simulink model "SVPWMtrialsyedek"  (R2015b)
settings: Solver=VariableStepAuto  StartTime=0.0  StopTime=1  RelTol=1e-3
libraries: powerlib x1
(part 1 of 2)
settings Model: Creator=hakan  LastModifiedBy=hakan

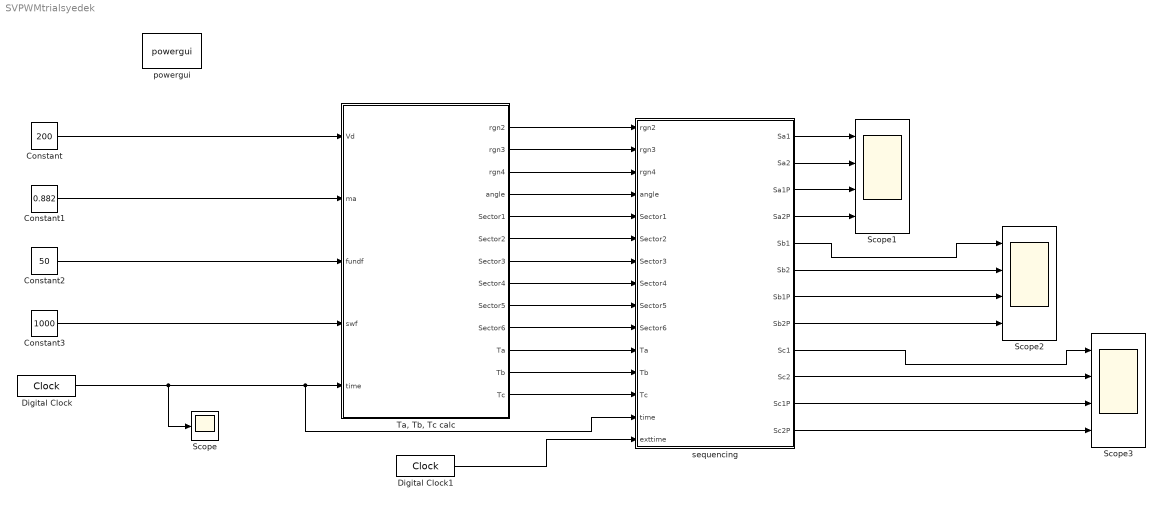
== system SVPWMtrialsyedek ==
  Constant : Constant  Value=200
  Constant1 : Constant  Value=0.882
  Constant2 : Constant  Value=50
  Constant3 : Constant  Value=1000
  Digital Clock : DigitalClock  SampleTime=0.001
  Digital Clock1 : DigitalClock  SampleTime=0.001
  Scope : Scope
  Scope1 : Scope  NumInputPorts=4
  Scope2 : Scope  NumInputPorts=4
  Scope3 : Scope  NumInputPorts=4
  "Ta, Tb, Tc calc" : MATLAB Function  TreatAsAtomicUnit=on
  powergui : powerlib/powergui  Priority=1  SimulationMode=Continuous  SolverType=Tustin/Backward Euler (TBE)  SampleTime=50e-6  frequency=60  SPID=off  DisableSnubberDevices=off  DisableRonSwitches=off  DisableVfSwitches=off  SwTol=0  DisplayEquations=off  Interpol=off  ExternalGateDelay=off  methode=off  Ts=10  FunctionMessages=off  echomessages=off  HookPort=off  EnableUseOfTLC=off  x0status=blocks  frequencyindice=60  Pbase=100e6  ErrMax=1e-4  Iterations=50  UnitsV=kV  UnitsW=MW  buscounter=0  RestoreLinks=warning  ResistiveCurrentMeasurement=off  Frange=[0:2:500]  Ylog=off  Xlog=on  ShowGrid=off  save=off  variable=ZData  structure=dutycycles  ZoomFFT=off  StartTime=0.0  cycles=1  DisplayStyle=1  fundamental=5000  FreqAxis=off  MaxFrequency=10000  frequencyindicesteady=1  RmsSteady=1  display=off
  sequencing : MATLAB Function  TreatAsAtomicUnit=on
  wires:
  Constant/1 -> "Ta, Tb, Tc calc"/1(Vd)
  Constant1/1 -> "Ta, Tb, Tc calc"/2(ma)
  Constant2/1 -> "Ta, Tb, Tc calc"/3(fundf)
  Constant3/1 -> "Ta, Tb, Tc calc"/4(swf)
  Digital Clock/1 -> sequencing/14(time), "Ta, Tb, Tc calc"/5(time), Scope/1
  "Ta, Tb, Tc calc"/1(rgn2) -> sequencing/1(rgn2)
  "Ta, Tb, Tc calc"/2(rgn3) -> sequencing/2(rgn3)
  "Ta, Tb, Tc calc"/3(rgn4) -> sequencing/3(rgn4)
  "Ta, Tb, Tc calc"/4(angle) -> sequencing/4(angle)
  "Ta, Tb, Tc calc"/5(Sector1) -> sequencing/5(Sector1)
  "Ta, Tb, Tc calc"/6(Sector2) -> sequencing/6(Sector2)
  "Ta, Tb, Tc calc"/7(Sector3) -> sequencing/7(Sector3)
  "Ta, Tb, Tc calc"/8(Sector4) -> sequencing/8(Sector4)
  "Ta, Tb, Tc calc"/10(Sector6) -> sequencing/10(Sector6)
  "Ta, Tb, Tc calc"/9(Sector5) -> sequencing/9(Sector5)
  "Ta, Tb, Tc calc"/11(Ta) -> sequencing/11(Ta)
  "Ta, Tb, Tc calc"/12(Tb) -> sequencing/12(Tb)
  "Ta, Tb, Tc calc"/13(Tc) -> sequencing/13(Tc)
  Digital Clock1/1 -> sequencing/15(exttime)
  sequencing/2(Sa2) -> Scope1/2
  sequencing/1(Sa1) -> Scope1/1
  sequencing/3(Sa1P) -> Scope1/3
  sequencing/4(Sa2P) -> Scope1/4
  sequencing/5(Sb1) -> Scope2/1
  sequencing/6(Sb2) -> Scope2/2
  sequencing/7(Sb1P) -> Scope2/3
  sequencing/8(Sb2P) -> Scope2/4
  sequencing/10(Sc2) -> Scope3/2
  sequencing/11(Sc1P) -> Scope3/3
  sequencing/12(Sc2P) -> Scope3/4
  sequencing/9(Sc1) -> Scope3/1

== matlab function SVPWMtrialsyedek/Ta, Tb, Tc calc ==
  data: rgn2 output; rgn3 output; rgn4 output; Vd input; ma input; fundf input; angle output; swf input; time input; Sector1 output; Sector2 output; Sector3 output; Sector4 output; Sector5 output; Sector6 output; Ta output; Tb output; Tc output
function [rgn2, rgn3, rgn4, angle, Sector1, Sector2, Sector3, Sector4, Sector5,Sector6, Ta, Tb, Tc] = fcn(Vd,ma,fundf, swf, time)
% this program works for magnitude of Vref is greater then Vd/3 meaning ma
% must be greater than 1/sqrt(3). for smaller ma's computation is a bit
% more tricky therefore it is omitted for simplicity for now. 
%#ok<*NASGU>
Vref = ma*Vd/sqrt(3); %magnitude of Vref
theta = 2*pi*fundf*time; %angle of Vref
angle = mod(theta, 2*pi);
Ts = 1/swf;
Ta = 0;
Tb = 0;
Tc = 0;
output = 0;
Sector1 = 0; Sector2 = 0; Sector3 = 0; Sector4= 0; Sector5 = 0; Sector6 = 0;
rgn2 = 0 ; rgn3 = 0; rgn4 = 0;
Sa1=0; Sa2=0; Sa1P=0; Sa2P=0; Sb1=0; Sb2=0; Sb1P=0; Sb2P=0; Sc1=0; Sc2=0; Sc1P=0; Sc2P=0;
%% Sector 1


if (mod(theta, 2*pi)<=pi/3)&&(mod(theta, 2*pi)>=0)  % sector 1

    n = 1;
    thetaprime = theta - (n-1)*pi/3;
    anglefrom3to2 = asin(1-1/(sqrt(3)*ma)); %leaving angle from region 3 to region 2
    anglefrom2to4 = pi/3 - anglefrom3to2; %leaving angle from region 2 to region 4
    if (mod(theta, 2*pi)<=anglefrom3to2) % then sector 1 region 3
        rgn3 = 1; rgn2= 0; rgn4=0;
        Ta = Ts*(2-2*ma*sin(pi/3+thetaprime));
        Tb = Ts*2*ma*sin(thetaprime);
        Tc = Ts*(2*ma*sin(pi/3-thetaprime)-1);        
    else if (mod(theta,2*pi)>=anglefrom3to2)&&(mod(theta,2*pi)<=anglefrom2to4) % then sector 1 region 2
            rgn3 = 0; rgn2= 1; rgn4=0;
            Ta = Ts*(1-2*ma*sin(thetaprime));
            Tb = Ts*(2*ma*sin(pi/3+thetaprime)-1);
            Tc = Ts*(1-2*ma*sin(pi/3-thetaprime));       
        else if (mod(theta,2*pi)>=anglefrom2to4) % then sector 1 region 4
               rgn3 = 0; rgn2= 0; rgn4=1;
               Ta = Ts*(2*ma*sin(thetaprime)-1);
               Tb = Ts*(2*ma*sin(pi/3-thetaprime));
               Tc = Ts*(2-2*ma*sin(pi/3+thetaprime));               
            end
        end
    end
    Sector1 = 1; Sector2 = 0; Sector3 = 0; Sector4= 0; Sector5 = 0; Sector6 = 0;
end
%% Sector 2


if (mod(theta, 2*pi)<=2*pi/3)&&(mod(theta, 2*pi)>=pi/3)  % sector 2
    
    n = 2;
    thetaprime = theta - (n-1)*pi/3;
    anglefrom3to2 = pi/3 + asin(1-1/(sqrt(3)*ma));
    anglefrom2to4 = pi/3 + pi/3 - anglefrom3to2;
    if (mod(theta, 2*pi)<=anglefrom3to2) % then sector 2 region 3
        rgn3 = 1; rgn2= 0; rgn4=0;
        Ta = Ts*(2-2*ma*sin(pi/3+thetaprime));
        Tb = Ts*2*ma*sin(thetaprime);
        Tc = Ts*(2*ma*sin(pi/3-thetaprime)-1); 
    else if (mod(theta,2*pi)>=anglefrom3to2)&&(mod(theta,2*pi)<=anglefrom2to4) % then sector 2 region 2
            rgn3 = 0; rgn2= 1; rgn4=0;
            Ta = Ts*(1-2*ma*sin(thetaprime));
            Tb = Ts*(2*ma*sin(pi/3+thetaprime)-1);
            Tc = Ts*(1-2*ma*sin(pi/3-thetaprime)); 
        else if (mod(theta,2*pi)>=anglefrom2to4) % then sector 2 region 4
               rgn3 = 0; rgn2= 0; rgn4=1;
               Ta = Ts*(2*ma*sin(thetaprime)-1);
               Tb = Ts*(2*ma*sin(pi/3-thetaprime));
               Tc = Ts*(2-2*ma*sin(pi/3+thetaprime)); 
            end
        end
    end
    Sector1 = 0; Sector2 = 1; Sector3 = 0; Sector4= 0; Sector5 = 0; Sector6 = 0;
end
%% Sector 3

if (mod(theta, 2*pi)<=pi)&&(mod(theta, 2*pi)>=2*pi/3)  % sector 3
    
    n = 3;
    thetaprime = theta - (n-1)*pi/3;
    anglefrom3to2 = 2*pi/3 + asin(1-1/(sqrt(3)*ma));
    anglefrom2to4 = 2*pi/3 + pi/3 - anglefrom3to2;
    if (mod(theta, 2*pi)<=anglefrom3to2) % then sector 3 region 3
        rgn3 = 1; rgn2= 0; rgn4=0;
        Ta = Ts*(2-2*ma*sin(pi/3+thetaprime));
        Tb = Ts*2*ma*sin(thetaprime);
        Tc = Ts*(2*ma*sin(pi/3-thetaprime)-1); 
    else if (mod(theta,2*pi)>=anglefrom3to2)&&(mod(theta,2*pi)<=anglefrom2to4) % then sector 3 region 2
            rgn3 = 0; rgn2= 1; rgn4=0;
            Ta = Ts*(1-2*ma*sin(thetaprime));
            Tb = Ts*(2*ma*sin(pi/3+thetaprime)-1);
            Tc = Ts*(1-2*ma*sin(pi/3-thetaprime)); 
        else if (mod(theta,2*pi)>=anglefrom2to4) % then sector 3 region 4
                rgn3 = 0; rgn2= 0; rgn4=1;
               Ta = Ts*(2*ma*sin(thetaprime)-1);
               Tb = Ts*(2*ma*sin(pi/3-thetaprime));
               Tc = Ts*(2-2*ma*sin(pi/3+thetaprime)); 
            end
        end
    end
    Sector1 = 0; Sector2 = 0; Sector3 = 1; Sector4= 0; Sector5 = 0; Sector6 = 0;
end

%% Sector 4


if (mod(theta, 2*pi)<=4*pi/3)&&(mod(theta, 2*pi)>=pi)  % sector 4
    

    n = 4;
    thetaprime = theta - (n-1)*pi/3;
    anglefrom3to2 = pi + asin(1-1/(sqrt(3)*ma));
    anglefrom2to4 = pi + pi/3 - anglefrom3to2;
    if (mod(theta, 2*pi)<=anglefrom3to2) % then sector 4 region 3
        rgn3 = 1; rgn2= 0; rgn4=0;
        Ta = Ts*(2-2*ma*sin(pi/3+thetaprime));
        Tb = Ts*2*ma*sin(thetaprime);
        Tc = Ts*(2*ma*sin(pi/3-thetaprime)-1); 
    else if (mod(theta,2*pi)>=anglefrom3to2)&&(mod(theta,2*pi)<=anglefrom2to4) % then sector 4 region 2
            rgn3 = 0; rgn2= 1; rgn4=0;
            Ta = Ts*(1-2*ma*sin(thetaprime));
            Tb = Ts*(2*ma*sin(pi/3+thetaprime)-1);
            Tc = Ts*(1-2*ma*sin(pi/3-thetaprime));
        else if (mod(theta,2*pi)>=anglefrom2to4) % then sector 4 region 4
                rgn3 = 0; rgn2= 0; rgn4=1;
               Ta = Ts*(2*ma*sin(thetaprime)-1);
               Tb = Ts*(2*ma*sin(pi/3-thetaprime));
               Tc = Ts*(2-2*ma*sin(pi/3+thetaprime)); 
            end
        end
    end
    Sector1 = 0; Sector2 = 0; Sector3 = 0; Sector4= 1; Sector5 = 0; Sector6 = 0;
end
%% Sector 5 

if (mod(theta, 2*pi)<=5*pi/3)&&(mod(theta, 2*pi)>=4*pi/3)  % sector 5
    
    n = 5;
    thetaprime = theta - (n-1)*pi/3;
    anglefrom3to2 = 4*pi/3 + asin(1-1/(sqrt(3)*ma));
    anglefrom2to4 = 4*pi/3 + pi/3 - anglefrom3to2;
    if (mod(theta, 2*pi)<=anglefrom3to2) % then sector 5 region 3
        rgn3 = 1; rgn2= 0; rgn4=0;
        Ta = Ts*(2-2*ma*sin(pi/3+thetaprime));
        Tb = Ts*2*ma*sin(thetaprime);
        Tc = Ts*(2*ma*sin(pi/3-thetaprime)-1); 
    else if (mod(theta,2*pi)>=anglefrom3to2)&&(mod(theta,2*pi)<=anglefrom2to4) % then sector 5 region 2
            rgn3 = 0; rgn2= 1; rgn4=0;
            Ta = Ts*(1-2*ma*sin(thetaprime));
            Tb = Ts*(2*ma*sin(pi/3+thetaprime)-1);
            Tc = Ts*(1-2*ma*sin(pi/3-thetaprime));
        else if (mod(theta,2*pi)>=anglefrom2to4) % then sector 5 region 4
               rgn3 = 0; rgn2= 0; rgn4=1;
               Ta = Ts*(2*ma*sin(thetaprime)-1);
               Tb = Ts*(2*ma*sin(pi/3-thetaprime));
               Tc = Ts*(2-2*ma*sin(pi/3+thetaprime)); 
            end
        end
    end
    Sector1 = 0; Sector2 = 0; Sector3 = 0; Sector4= 0; Sector5 = 1; Sector6 = 0;
end

%% Sector 6 

if (mod(theta, 2*pi)<=2*pi)&&(mod(theta, 2*pi)>=5*pi/3)  % sector 6
    
    n = 6;
    thetaprime = theta - (n-1)*pi/3;
    anglefrom3to2 = 5*pi/3 + asin(1-1/(sqrt(3)*ma));
    anglefrom2to4 = 5*pi/3 + pi/3 - anglefrom3to2;
    if (mod(theta, 2*pi)<=anglefrom3to2) % then sector 6 region 3
        rgn3 = 1; rgn2= 0; rgn4=0;
        Ta = Ts*(2-2*ma*sin(pi/3+thetaprime));
        Tb = Ts*2*ma*sin(thetaprime);
        Tc = Ts*(2*ma*sin(pi/3-thetaprime)-1); 
    else if (mod(theta,2*pi)>=anglefrom3to2)&&(mod(theta,2*pi)<=anglefrom2to4) % then sector 6 region 2
            rgn3 = 0; rgn2= 1; rgn4=0;
            Ta = Ts*(1-2*ma*sin(thetaprime));
            Tb = Ts*(2*ma*sin(pi/3+thetaprime)-1);
            Tc = Ts*(1-2*ma*sin(pi/3-thetaprime));
        else if (mod(theta,2*pi)>=anglefrom2to4) % then sector 6 region 4
               rgn3 = 0; rgn2= 0; rgn4=1;
               Ta = Ts*(2*ma*sin(thetaprime)-1);
               Tb = Ts*(2*ma*sin(pi/3-thetaprime));
               Tc = Ts*(2-2*ma*sin(pi/3+thetaprime)); 
            end
        end
    end
    Sector1 = 0; Sector2 = 0; Sector3 = 0; Sector4= 0; Sector5 = 0; Sector6 = 1;
end
%% Sequencing Part
% while(Sector1)
%     while(rgn3)
%         Sa1=0; Sa2=1; Sa1P=1; Sa2P=0;
%         Sb1=0; Sb2=0; Sb1P=1; Sb2P=1; 
%         Sc1=0; Sc2=0; Sc1P=1; Sc2P=1;
%         pause(Tc/4);
%         Sa1=1; Sa2=1; Sa1P=0; Sa2P=0;
%         Sb1=0; Sb2=0; Sb1P=1; Sb2P=1; 
%         Sc1=0; Sc2=0; Sc1P=1; Sc2P=1;
%         pause(Tb/2);
%         Sa1=1; Sa2=1; Sa1P=0; Sa2P=0;
%         Sb1=0; Sb2=1; Sb1P=1; Sb2P=0; 
%         Sc1=0; Sc2=0; Sc1P=1; Sc2P=1;
%         pause(Ta/2);
%         Sa1=1; Sa2=1; Sa1P=0; Sa2P=0;
%         Sb1=0; Sb2=1; Sb1P=1; Sb2P=0; 
%         Sc1=0; Sc2=1; Sc1P=1; Sc2P=0;
%         pause(Tc/2);
%         Sa1=1; Sa2=1; Sa1P=0; Sa2P=0;
%         Sb1=0; Sb2=1; Sb1P=1; Sb2P=0; 
%         Sc1=0; Sc2=0; Sc1P=1; Sc2P=1;
%         pause(Ta/2);
%         Sa1=1; Sa2=1; Sa1P=0; Sa2P=0;
%         Sb1=0; Sb2=0; Sb1P=1; Sb2P=1; 
%         Sc1=0; Sc2=0; Sc1P=1; Sc2P=1;
%         pause(Tb/2);
%         Sa1=0; Sa2=1; Sa1P=1; Sa2P=0;
%         Sb1=0; Sb2=0; Sb1P=1; Sb2P=1; 
%         Sc1=0; Sc2=0; Sc1P=1; Sc2P=1;
%         pause(Tc/4);        
%     end
%     while(rgn2)
%         if angle<= pi/6 % then 2a
%             Sa1=0; Sa2=1; Sa1P=1; Sa2P=0;
%             Sb1=0; Sb2=0; Sb1P=1; Sb2P=1; 
%             Sc1=0; Sc2=0; Sc1P=1; Sc2P=1;
%             pause(Tc/4);
%             Sa1=0; Sa2=1; Sa1P=1; Sa2P=0;
%             Sb1=0; Sb2=1; Sb1P=1; Sb2P=0; 
%             Sc1=0; Sc2=0; Sc1P=1; Sc2P=1;
%             pause(Tb/2);
%             Sa1=1; Sa2=1; Sa1P=0; Sa2P=0;
%             Sb1=0; Sb2=1; Sb1P=1; Sb2P=0; 
%             Sc1=0; Sc2=0; Sc1P=1; Sc2P=1;       
%             pause(Ta/2);
%             Sa1=1; Sa2=1; Sa1P=0; Sa2P=0;
%             Sb1=0; Sb2=1; Sb1P=1; Sb2P=0; 
%             Sc1=0; Sc2=1; Sc1P=1; Sc2P=0;
%             pause(Tc/2);
%             Sa1=1; Sa2=1; Sa1P=0; Sa2P=0;
%             Sb1=0; Sb2=1; Sb1P=1; Sb2P=0; 
%             Sc1=0; Sc2=0; Sc1P=1; Sc2P=1;
%             pause(Ta/2);
%             Sa1=0; Sa2=1; Sa1P=1; Sa2P=0;
%             Sb1=0; Sb2=1; Sb1P=1; Sb2P=0; 
%             Sc1=0; Sc2=0; Sc1P=1; Sc2P=1;
%             pause(Tb/2);
%             Sa1=0; Sa2=1; Sa1P=1; Sa2P=0;
%             Sb1=0; Sb2=0; Sb1P=1; Sb2P=1; 
%             Sc1=0; Sc2=0; Sc1P=1; Sc2P=1;
%             pause(Tc/4);        
%         end
%         if angle>= pi/6 % then 2b
%             Sa1=0; Sa2=1; Sa1P=1; Sa2P=0;
%             Sb1=0; Sb2=1; Sb1P=1; Sb2P=0; 
%             Sc1=0; Sc2=0; Sc1P=1; Sc2P=1;
%             pause(Tc/4);
%             Sa1=1; Sa2=1; Sa1P=0; Sa2P=0;
%             Sb1=0; Sb2=1; Sb1P=1; Sb2P=0; 
%             Sc1=0; Sc2=0; Sc1P=1; Sc2P=1;
%             pause(Tb/2);
%             Sa1=1; Sa2=1; Sa1P=0; Sa2P=0;
%             Sb1=0; Sb2=1; Sb1P=1; Sb2P=0; 
%             Sc1=0; Sc2=1; Sc1P=1; Sc2P=0;
%             pause(Ta/2);
%             Sa1=1; Sa2=1; Sa1P=0; Sa2P=0;
%             Sb1=1; Sb2=1; Sb1P=0; Sb2P=0; 
%             Sc1=0; Sc2=1; Sc1P=1; Sc2P=0;
%             pause(Tc/2);
%             Sa1=1; Sa2=1; Sa1P=0; Sa2P=0;
%             Sb1=0; Sb2=1; Sb1P=1; Sb2P=0; 
%             Sc1=0; Sc2=1; Sc1P=1; Sc2P=0;
%             pause(Ta/2);
%             Sa1=1; Sa2=1; Sa1P=0; Sa2P=0;
%             Sb1=0; Sb2=1; Sb1P=1; Sb2P=0; 
%             Sc1=0; Sc2=0; Sc1P=1; Sc2P=1;
%             pause(Tb/2);
%             Sa1=0; Sa2=1; Sa1P=1; Sa2P=0;
%             Sb1=0; Sb2=1; Sb1P=1; Sb2P=0; 
%             Sc1=0; Sc2=0; Sc1P=1; Sc2P=1;
%             pause(Tc/4);
%         end
%     end
%     while(rgn4)
%         Sa1=0; Sa2=1; Sa1P=1; Sa2P=0;
%         Sb1=0; Sb2=1; Sb1P=1; Sb2P=0;
%         Sc1=0; Sc2=0; Sc1P=1; Sc2P=1;
%         pause(Tc/4);
%         Sa1=1; Sa2=1; Sa1P=0; Sa2P=0;
%         Sb1=0; Sb2=1; Sb1P=1; Sb2P=0;
%         Sc1=0; Sc2=0; Sc1P=1; Sc2P=1;        
%         pause(Tb/2);        
%         Sa1=1; Sa2=1; Sa1P=0; Sa2P=0;
%         Sb1=1; Sb2=1; Sb1P=0; Sb2P=0;
%         Sc1=0; Sc2=0; Sc1P=1; Sc2P=1;
%         pause(Ta/2);
%         Sa1=1; Sa2=1; Sa1P=0; Sa2P=0;
%         Sb1=1; Sb2=1; Sb1P=0; Sb2P=0;
%         Sc1=0; Sc2=1; Sc1P=1; Sc2P=0;
%         pause(Tc/2);
%         Sa1=1; Sa2=1; Sa1P=0; Sa2P=0;
%         Sb1=1; Sb2=1; Sb1P=0; Sb2P=0;
%         Sc1=0; Sc2=0; Sc1P=1; Sc2P=1;
%         pause(Ta/2);        
%         Sa1=1; Sa2=1; Sa1P=0; Sa2P=0;
%         Sb1=0; Sb2=1; Sb1P=1; Sb2P=0;
%         Sc1=0; Sc2=0; Sc1P=1; Sc2P=1;        
%         pause(Tb/2);
%         Sa1=0; Sa2=1; Sa1P=1; Sa2P=0;
%         Sb1=0; Sb2=1; Sb1P=1; Sb2P=0;
%         Sc1=0; Sc2=0; Sc1P=1; Sc2P=1;
%         pause(Tc/4);
%     end
% end
% while(Sector2)
%     while(rgn3)        
%         Sa1=0; Sa2=1; Sa1P=1; Sa2P=0;
%         Sb1=0; Sb2=1; Sb1P=1; Sb2P=0;
%         Sc1=0; Sc2=0; Sc1P=1; Sc2P=1;
%         pause(Tc/4);
%         Sa1=0; Sa2=1; Sa1P=1; Sa2P=0;
%         Sb1=1; Sb2=1; Sb1P=0; Sb2P=0;
%         Sc1=0; Sc2=0; Sc1P=1; Sc2P=1;
%         pause(Tb/2);
%         Sa1=1; Sa2=1; Sa1P=0; Sa2P=0;
%         Sb1=1; Sb2=1; Sb1P=0; Sb2P=0;
%         Sc1=0; Sc2=0; Sc1P=1; Sc2P=1;
%         pause(Ta/2);
%         Sa1=1; Sa2=1; Sa1P=0; Sa2P=0;
%         Sb1=1; Sb2=1; Sb1P=0; Sb2P=0;
%         Sc1=0; Sc2=1; Sc1P=1; Sc2P=0;       
%         pause(Tc/2);
%         Sa1=1; Sa2=1; Sa1P=0; Sa2P=0;
%         Sb1=1; Sb2=1; Sb1P=0; Sb2P=0;
%         Sc1=0; Sc2=0; Sc1P=1; Sc2P=1;
%         pause(Ta/2);
%         Sa1=0; Sa2=1; Sa1P=1; Sa2P=0;
%         Sb1=1; Sb2=1; Sb1P=0; Sb2P=0;
%         Sc1=0; Sc2=0; Sc1P=1; Sc2P=1;
%         pause(Tb/2);
%         Sa1=0; Sa2=1; Sa1P=1; Sa2P=0;
%         Sb1=0; Sb2=1; Sb1P=1; Sb2P=0;
%         Sc1=0; Sc2=0; Sc1P=1; Sc2P=1;
%         pause(Tc/4);       
%     end
%     while(rgn2)
%         if angle<=pi/2 %then 2a
%             Sa1=0; Sa2=1; Sa1P=1; Sa2P=0;
%             Sb1=0; Sb2=1; Sb1P=1; Sb2P=0;
%             Sc1=0; Sc2=0; Sc1P=1; Sc2P=1;
%             pause(Tc/4);
%             Sa1=0; Sa2=1; Sa1P=1; Sa2P=0;
%             Sb1=1; Sb2=1; Sb1P=0; Sb2P=0;
%             Sc1=0; Sc2=0; Sc1P=1; Sc2P=1;
%             pause(Tb/2);
%             Sa1=0; Sa2=1; Sa1P=1; Sa2P=0;
%             Sb1=1; Sb2=1; Sb1P=0; Sb2P=0;
%             Sc1=0; Sc2=1; Sc1P=1; Sc2P=0;
%             pause(Ta/2);
%             Sa1=1; Sa2=1; Sa1P=0; Sa2P=0;
%             Sb1=1; Sb2=1; Sb1P=0; Sb2P=0;
%             Sc1=0; Sc2=1; Sc1P=1; Sc2P=0;            
%             pause(Tc/2);
%             Sa1=0; Sa2=1; Sa1P=1; Sa2P=0;
%             Sb1=1; Sb2=1; Sb1P=0; Sb2P=0;
%             Sc1=0; Sc2=1; Sc1P=1; Sc2P=0;
%             pause(Ta/2);
%             Sa1=0; Sa2=1; Sa1P=1; Sa2P=0;
%             Sb1=1; Sb2=1; Sb1P=0; Sb2P=0;
%             Sc1=0; Sc2=0; Sc1P=1; Sc2P=1;
%             pause(Tb/2);
%             Sa1=0; Sa2=1; Sa1P=1; Sa2P=0;
%             Sb1=0; Sb2=1; Sb1P=1; Sb2P=0;
%             Sc1=0; Sc2=0; Sc1P=1; Sc2P=1;
%             pause(Tc/4);
%         end
%         if angle>=pi/2 %then 2b
%             Sa1=0; Sa2=0; Sa1P=1; Sa2P=1;
%             Sb1=0; Sb2=1; Sb1P=1; Sb2P=0;
%             Sc1=0; Sc2=0; Sc1P=1; Sc2P=1;
%             pause(Tc/4);
%             Sa1=0; Sa2=1; Sa1P=1; Sa2P=0;
%             Sb1=0; Sb2=1; Sb1P=1; Sb2P=0;
%             Sc1=0; Sc2=0; Sc1P=1; Sc2P=1;
%             pause(Tb/2);
%             Sa1=0; Sa2=1; Sa1P=1; Sa2P=0;
%             Sb1=1; Sb2=1; Sb1P=0; Sb2P=0;
%             Sc1=0; Sc2=0; Sc1P=1; Sc2P=1;
%             pause(Ta/2);
%             Sa1=0; Sa2=1; Sa1P=1; Sa2P=0;
%             Sb1=1; Sb2=1; Sb1P=0; Sb2P=0;
%             Sc1=0; Sc2=1; Sc1P=1; Sc2P=0;
%             pause(Tc/2);
%             Sa1=0; Sa2=1; Sa1P=1; Sa2P=0;
%             Sb1=1; Sb2=1; Sb1P=0; Sb2P=0;
%             Sc1=0; Sc2=0; Sc1P=1; Sc2P=1;
%             pause(Ta/2);
%             Sa1=0; Sa2=1; Sa1P=1; Sa2P=0;
%             Sb1=0; Sb2=1; Sb1P=1; Sb2P=0;
%             Sc1=0; Sc2=0; Sc1P=1; Sc2P=1;
%             pause(Tb/2);
%             Sa1=0; Sa2=0; Sa1P=1; Sa2P=1;
%             Sb1=0; Sb2=1; Sb1P=1; Sb2P=0;
%             Sc1=0; Sc2=0; Sc1P=1; Sc2P=1;
%             pause(Tc/4);           
%         end
%     end
%     while(rgn4)
%         Sa1=0; Sa2=0; Sa1P=1; Sa2P=1;
%         Sb1=0; Sb2=1; Sb1P=1; Sb2P=0;
%         Sc1=0; Sc2=0; Sc1P=1; Sc2P=1;
%         pause(Tc/4);
%         Sa1=0; Sa2=0; Sa1P=1; Sa2P=1;
%         Sb1=1; Sb2=1; Sb1P=0; Sb2P=0;
%         Sc1=0; Sc2=0; Sc1P=1; Sc2P=1;
%         pause(Tb/2);
%         Sa1=0; Sa2=1; Sa1P=1; Sa2P=0;
%         Sb1=1; Sb2=1; Sb1P=0; Sb2P=0;
%         Sc1=0; Sc2=0; Sc1P=1; Sc2P=1;
%         pause(Ta/2);
%         Sa1=0; Sa2=1; Sa1P=1; Sa2P=0;
%         Sb1=1; Sb2=1; Sb1P=0; Sb2P=0;
%         Sc1=0; Sc2=1; Sc1P=1; Sc2P=0;
%         pause(Tc/2); 
%         Sa1=0; Sa2=1; Sa1P=1; Sa2P=0;
%         Sb1=1; Sb2=1; Sb1P=0; Sb2P=0;
%         Sc1=0; Sc2=0; Sc1P=1; Sc2P=1;
%         pause(Ta/2);
%         Sa1=0; Sa2=0; Sa1P=1; Sa2P=1;
%         Sb1=1; Sb2=1; Sb1P=0; Sb2P=0;
%         Sc1=0; Sc2=0; Sc1P=1; Sc2P=1;
%         pause(Tb/2);
%         Sa1=0; Sa2=0; Sa1P=1; Sa2P=1;
%         Sb1=0; Sb2=1; Sb1P=1; Sb2P=0;
%         Sc1=0; Sc2=0; Sc1P=1; Sc2P=1;
%         pause(Tc/4);
%         
%     end
% 
% end
% while(Sector3)
%     while(rgn3)
%         Sa1=0; Sa2=0; Sa1P=1; Sa2P=1;
%         Sb1=0; Sb2=1; Sb1P=1; Sb2P=0;
%         Sc1=0; Sc2=0; Sc1P=1; Sc2P=1;
%         pause(Tc/4);
%         Sa1=0; Sa2=0; Sa1P=1; Sa2P=1;
%         Sb1=1; Sb2=1; Sb1P=0; Sb2P=0;
%         Sc1=0; Sc2=0; Sc1P=1; Sc2P=1;
%         pause(Tb/2);
%         Sa1=0; Sa2=0; Sa1P=1; Sa2P=1;
%         Sb1=1; Sb2=1; Sb1P=0; Sb2P=0;
%         Sc1=0; Sc2=1; Sc1P=1; Sc2P=0;
%         pause(Ta/2);
%         Sa1=0; Sa2=1; Sa1P=1; Sa2P=0;
%         Sb1=1; Sb2=1; Sb1P=0; Sb2P=0;
%         Sc1=0; Sc2=1; Sc1P=1; Sc2P=0;
%         pause(Tc/2);
%         Sa1=0; Sa2=0; Sa1P=1; Sa2P=1;
%         Sb1=1; Sb2=1; Sb1P=0; Sb2P=0;
%         Sc1=0; Sc2=1; Sc1P=1; Sc2P=0;
%         pause(Ta/2);
%         Sa1=0; Sa2=0; Sa1P=1; Sa2P=1;
%         Sb1=1; Sb2=1; Sb1P=0; Sb2P=0;
%         Sc1=0; Sc2=0; Sc1P=1; Sc2P=1;
%         pause(Tb/2);
%         Sa1=0; Sa2=0; Sa1P=1; Sa2P=1;
%         Sb1=0; Sb2=1; Sb1P=1; Sb2P=0;
%         Sc1=0; Sc2=0; Sc1P=1; Sc2P=1;
%         pause(Tc/4);        
%     end
%     while(rgn2)
%         if angle<=5*pi/6 %then 2a
%             Sa1=0; Sa2=0; Sa1P=1; Sa2P=1;
%             Sb1=0; Sb2=1; Sb1P=1; Sb2P=0;
%             Sc1=0; Sc2=0; Sc1P=1; Sc2P=1;
%             pause(Tc/4);
%             Sa1=0; Sa2=0; Sa1P=1; Sa2P=1;
%             Sb1=0; Sb2=1; Sb1P=1; Sb2P=0;
%             Sc1=0; Sc2=1; Sc1P=1; Sc2P=0;
%             pause(Tb/2);
%             Sa1=0; Sa2=0; Sa1P=1; Sa2P=1;
%             Sb1=1; Sb2=1; Sb1P=0; Sb2P=0;
%             Sc1=0; Sc2=1; Sc1P=1; Sc2P=0;
%             pause(Ta/2);
%             Sa1=0; Sa2=0; Sa1P=1; Sa2P=1;
%             Sb1=1; Sb2=1; Sb1P=0; Sb2P=0;
%             Sc1=0; Sc2=0; Sc1P=1; Sc2P=1;
%             pause(Tc/2);
%             Sa1=0; Sa2=0; Sa1P=1; Sa2P=1;
%             Sb1=1; Sb2=1; Sb1P=0; Sb2P=0;
%             Sc1=0; Sc2=1; Sc1P=1; Sc2P=0;
%             pause(Ta/2);
%             Sa1=0; Sa2=0; Sa1P=1; Sa2P=1;
%             Sb1=0; Sb2=1; Sb1P=1; Sb2P=0;
%             Sc1=0; Sc2=1; Sc1P=1; Sc2P=0;
%             pause(Tb/2);
%             Sa1=0; Sa2=0; Sa1P=1; Sa2P=1;
%             Sb1=0; Sb2=1; Sb1P=1; Sb2P=0;
%             Sc1=0; Sc2=0; Sc1P=1; Sc2P=1;
%             pause(Tc/4);           
%         end
%         if angle>=5*pi/6 %then 2b
%             Sa1=0; Sa2=0; Sa1P=1; Sa2P=1;
%             Sb1=0; Sb2=1; Sb1P=1; Sb2P=0;
%             Sc1=0; Sc2=1; Sc1P=1; Sc2P=0;
%             pause(Tc/4);
%             Sa1=0; Sa2=0; Sa1P=1; Sa2P=1;
%             Sb1=1; Sb2=1; Sb1P=0; Sb2P=0;
%             Sc1=0; Sc2=1; Sc1P=1; Sc2P=0;
%             pause(Tb/2);
%             Sa1=0; Sa2=1; Sa1P=1; Sa2P=0;
%             Sb1=1; Sb2=1; Sb1P=0; Sb2P=0;
%             Sc1=0; Sc2=1; Sc1P=1; Sc2P=0;
%             pause(Ta/2);
%             Sa1=0; Sa2=1; Sa1P=1; Sa2P=0;
%             Sb1=1; Sb2=1; Sb1P=0; Sb2P=0;
%             Sc1=1; Sc2=1; Sc1P=0; Sc2P=0;
%             pause(Tc/2);
%             Sa1=0; Sa2=1; Sa1P=1; Sa2P=0;
%             Sb1=1; Sb2=1; Sb1P=0; Sb2P=0;
%             Sc1=0; Sc2=1; Sc1P=1; Sc2P=0;
%             pause(Ta/2);
%             Sa1=0; Sa2=0; Sa1P=1; Sa2P=1;
%             Sb1=1; Sb2=1; Sb1P=0; Sb2P=0;
%             Sc1=0; Sc2=1; Sc1P=1; Sc2P=0;
%             pause(Tb/2);
%             Sa1=0; Sa2=0; Sa1P=1; Sa2P=1;
%             Sb1=0; Sb2=1; Sb1P=1; Sb2P=0;
%             Sc1=0; Sc2=1; Sc1P=1; Sc2P=0;
%             pause(Tc/4);            
%         end
%     end
%     while(rgn4)
%         Sa1=0; Sa2=0; Sa1P=1; Sa2P=1;
%         Sb1=0; Sb2=1; Sb1P=1; Sb2P=0;
%         Sc1=0; Sc2=1; Sc1P=1; Sc2P=0;
%         pause(Tc/4);
%         Sa1=0; Sa2=0; Sa1P=1; Sa2P=1;
%         Sb1=1; Sb2=1; Sb1P=0; Sb2P=0;
%         Sc1=0; Sc2=1; Sc1P=1; Sc2P=0;
%         pause(Tb/2);
%         Sa1=0; Sa2=0; Sa1P=1; Sa2P=1;
%         Sb1=1; Sb2=1; Sb1P=0; Sb2P=0;
%         Sc1=1; Sc2=1; Sc1P=0; Sc2P=0;
%         pause(Ta/2);
%         Sa1=0; Sa2=1; Sa1P=1; Sa2P=0;
%         Sb1=1; Sb2=1; Sb1P=0; Sb2P=0;
%         Sc1=1; Sc2=1; Sc1P=0; Sc2P=0;
%         pause(Tc/2);
%         Sa1=0; Sa2=0; Sa1P=1; Sa2P=1;
%         Sb1=1; Sb2=1; Sb1P=0; Sb2P=0;
%         Sc1=1; Sc2=1; Sc1P=0; Sc2P=0;
%         pause(Ta/2);
%         Sa1=0; Sa2=0; Sa1P=1; Sa2P=1;
%         Sb1=1; Sb2=1; Sb1P=0; Sb2P=0;
%         Sc1=0; Sc2=1; Sc1P=1; Sc2P=0;
%         pause(Tb/2);
%         Sa1=0; Sa2=0; Sa1P=1; Sa2P=1;
%         Sb1=0; Sb2=1; Sb1P=1; Sb2P=0;
%         Sc1=0; Sc2=1; Sc1P=1; Sc2P=0;
%         pause(Tc/4);
%     end
% end
% while(Sector4)
%     while(rgn3)        
%         Sa1=0; Sa2=1; Sa1P=1; Sa2P=0;
%         Sb1=1; Sb2=1; Sb1P=0; Sb2P=0;
%         Sc1=1; Sc2=1; Sc1P=0; Sc2P=0;
%         pause(Tc/4);
%         Sa1=0; Sa2=0; Sa1P=1; Sa2P=1;
%         Sb1=1; Sb2=1; Sb1P=0; Sb2P=0;
%         Sc1=1; Sc2=1; Sc1P=0; Sc2P=0;
%         pause(Tb/2);
%         Sa1=0; Sa2=0; Sa1P=1; Sa2P=1;
%         Sb1=0; Sb2=1; Sb1P=1; Sb2P=0;
%         Sc1=1; Sc2=1; Sc1P=0; Sc2P=0;
%         pause(Ta/2);
%         Sa1=0; Sa2=0; Sa1P=1; Sa2P=1;
%         Sb1=0; Sb2=1; Sb1P=1; Sb2P=0;
%         Sc1=0; Sc2=1; Sc1P=1; Sc2P=0;
%         pause(Tc/2);
%         Sa1=0; Sa2=0; Sa1P=1; Sa2P=1;
%         Sb1=0; Sb2=1; Sb1P=1; Sb2P=0;
%         Sc1=1; Sc2=1; Sc1P=0; Sc2P=0;
%         pause(Ta/2);
%         Sa1=0; Sa2=0; Sa1P=1; Sa2P=1;
%         Sb1=1; Sb2=1; Sb1P=0; Sb2P=0;
%         Sc1=1; Sc2=1; Sc1P=0; Sc2P=0;
%         pause(Tb/2);
%         Sa1=0; Sa2=1; Sa1P=1; Sa2P=0;
%         Sb1=1; Sb2=1; Sb1P=0; Sb2P=0;
%         Sc1=1; Sc2=1; Sc1P=0; Sc2P=0;
%         pause(Tc/4);
%     end
%     while(rgn2)
%         if angle<=7*pi/6 %then 2a
%             Sa1=0; Sa2=1; Sa1P=1; Sa2P=0;
%             Sb1=1; Sb2=1; Sb1P=0; Sb2P=0;
%             Sc1=1; Sc2=1; Sc1P=0; Sc2P=0;
%             pause(Tc/4);
%             Sa1=0; Sa2=1; Sa1P=1; Sa2P=0;
%             Sb1=0; Sb2=1; Sb1P=1; Sb2P=0;
%             Sc1=1; Sc2=1; Sc1P=0; Sc2P=0;
%             pause(Tb/2);
%             Sa1=0; Sa2=0; Sa1P=1; Sa2P=1;
%             Sb1=0; Sb2=1; Sb1P=1; Sb2P=0;
%             Sc1=1; Sc2=1; Sc1P=0; Sc2P=0;
%             pause(Ta/2);
%             Sa1=0; Sa2=0; Sa1P=1; Sa2P=1;
%             Sb1=0; Sb2=1; Sb1P=1; Sb2P=0;
%             Sc1=0; Sc2=1; Sc1P=1; Sc2P=0;
%             pause(Tc/2);
%             Sa1=0; Sa2=0; Sa1P=1; Sa2P=1;
%             Sb1=0; Sb2=1; Sb1P=1; Sb2P=0;
%             Sc1=1; Sc2=1; Sc1P=0; Sc2P=0;
%             pause(Ta/2);
%             Sa1=0; Sa2=1; Sa1P=1; Sa2P=0;
%             Sb1=0; Sb2=1; Sb1P=1; Sb2P=0;
%             Sc1=1; Sc2=1; Sc1P=0; Sc2P=0;
%             pause(Tb/2);
%             Sa1=0; Sa2=1; Sa1P=1; Sa2P=0;
%             Sb1=1; Sb2=1; Sb1P=0; Sb2P=0;
%             Sc1=1; Sc2=1; Sc1P=0; Sc2P=0;
%             pause(Tc/4);           
%         end
%         if angle>=7*pi/6 %then 2b
%             Sa1=0; Sa2=1; Sa1P=1; Sa2P=0;
%             Sb1=0; Sb2=1; Sb1P=1; Sb2P=0;
%             Sc1=1; Sc2=1; Sc1P=0; Sc2P=0;
%             pause(Tc/4);
%             Sa1=0; Sa2=0; Sa1P=1; Sa2P=1;
%             Sb1=0; Sb2=1; Sb1P=1; Sb2P=0;
%             Sc1=1; Sc2=1; Sc1P=0; Sc2P=0;
%             pause(Tb/2);
%             Sa1=0; Sa2=0; Sa1P=1; Sa2P=1;
%             Sb1=0; Sb2=1; Sb1P=1; Sb2P=0;
%             Sc1=0; Sc2=1; Sc1P=1; Sc2P=0;
%             pause(Ta/2);
%             Sa1=0; Sa2=0; Sa1P=1; Sa2P=1;
%             Sb1=0; Sb2=0; Sb1P=1; Sb2P=1;
%             Sc1=0; Sc2=1; Sc1P=1; Sc2P=0;
%             pause(Tc/2);
%             Sa1=0; Sa2=0; Sa1P=1; Sa2P=1;
%             Sb1=0; Sb2=1; Sb1P=1; Sb2P=0;
%             Sc1=0; Sc2=1; Sc1P=1; Sc2P=0;
%             pause(Ta/2);
%             Sa1=0; Sa2=0; Sa1P=1; Sa2P=1;
%             Sb1=0; Sb2=1; Sb1P=1; Sb2P=0;
%             Sc1=1; Sc2=1; Sc1P=0; Sc2P=0;
%             pause(Tb/2);
%             Sa1=0; Sa2=1; Sa1P=1; Sa2P=0;
%             Sb1=0; Sb2=1; Sb1P=1; Sb2P=0;
%             Sc1=1; Sc2=1; Sc1P=0; Sc2P=0;
%             pause(Tc/4);                      
%         end
%     end
%     while(rgn4)
%         Sa1=0; Sa2=1; Sa1P=1; Sa2P=0;
%         Sb1=0; Sb2=1; Sb1P=1; Sb2P=0;
%         Sc1=1; Sc2=1; Sc1P=0; Sc2P=0;
%         pause(Tc/4);
%         Sa1=0; Sa2=0; Sa1P=1; Sa2P=1;
%         Sb1=0; Sb2=1; Sb1P=1; Sb2P=0;
%         Sc1=1; Sc2=1; Sc1P=0; Sc2P=0;
%         pause(Tb/2);
%         Sa1=0; Sa2=0; Sa1P=1; Sa2P=1;
%         Sb1=0; Sb2=0; Sb1P=1; Sb2P=1;
%         Sc1=1; Sc2=1; Sc1P=0; Sc2P=0;
%         pause(Ta/2);
%         Sa1=0; Sa2=0; Sa1P=1; Sa2P=1;
%         Sb1=0; Sb2=0; Sb1P=1; Sb2P=1;
%         Sc1=0; Sc2=1; Sc1P=1; Sc2P=0;
%         pause(Tc/2);
%         Sa1=0; Sa2=0; Sa1P=1; Sa2P=1;
%         Sb1=0; Sb2=0; Sb1P=1; Sb2P=1;
%         Sc1=1; Sc2=1; Sc1P=0; Sc2P=0;
%         pause(Ta/2);
%         Sa1=0; Sa2=0; Sa1P=1; Sa2P=1;
%         Sb1=0; Sb2=1; Sb1P=1; Sb2P=0;
%         Sc1=1; Sc2=1; Sc1P=0; Sc2P=0;
%         pause(Tb/2);
%         Sa1=0; Sa2=1; Sa1P=1; Sa2P=0;
%         Sb1=0; Sb2=1; Sb1P=1; Sb2P=0;
%         Sc1=1; Sc2=1; Sc1P=0; Sc2P=0;
%         pause(Tc/4);
%     end     
% end
% while(Sector5)
%     while(rgn3)
%         Sa1=0; Sa2=1; Sa1P=1; Sa2P=0;
%         Sb1=0; Sb2=1; Sb1P=1; Sb2P=0;
%         Sc1=1; Sc2=1; Sc1P=0; Sc2P=0;
%         pause(Tc/4);
%         Sa1=0; Sa2=1; Sa1P=1; Sa2P=0;
%         Sb1=0; Sb2=0; Sb1P=1; Sb2P=1;
%         Sc1=1; Sc2=1; Sc1P=0; Sc2P=0;
%         pause(Tb/2);
%         Sa1=0; Sa2=0; Sa1P=1; Sa2P=1;
%         Sb1=0; Sb2=0; Sb1P=1; Sb2P=1;
%         Sc1=1; Sc2=1; Sc1P=0; Sc2P=0;
%         pause(Ta/2);
%         Sa1=0; Sa2=0; Sa1P=1; Sa2P=1;
%         Sb1=0; Sb2=0; Sb1P=1; Sb2P=1;
%         Sc1=0; Sc2=1; Sc1P=1; Sc2P=0;
%         pause(Tc/2);
%         Sa1=0; Sa2=0; Sa1P=1; Sa2P=1;
%         Sb1=0; Sb2=0; Sb1P=1; Sb2P=1;
%         Sc1=1; Sc2=1; Sc1P=0; Sc2P=0;
%         pause(Ta/2);
%         Sa1=0; Sa2=1; Sa1P=1; Sa2P=0;
%         Sb1=0; Sb2=0; Sb1P=1; Sb2P=1;
%         Sc1=1; Sc2=1; Sc1P=0; Sc2P=0;
%         pause(Tb/2);
%         Sa1=0; Sa2=1; Sa1P=1; Sa2P=0;
%         Sb1=0; Sb2=1; Sb1P=1; Sb2P=0;
%         Sc1=1; Sc2=1; Sc1P=0; Sc2P=0;
%         pause(Tc/4);
%     end
%     while(rgn2)
%         if angle<=3*pi/2 %then 2a
%             Sa1=0; Sa2=1; Sa1P=1; Sa2P=0;
%             Sb1=0; Sb2=1; Sb1P=1; Sb2P=0;
%             Sc1=1; Sc2=1; Sc1P=0; Sc2P=0;
%             pause(Tc/4);
%             Sa1=0; Sa2=1; Sa1P=1; Sa2P=0;
%             Sb1=0; Sb2=0; Sb1P=1; Sb2P=1;
%             Sc1=1; Sc2=1; Sc1P=0; Sc2P=0;
%             pause(Tb/2);
%             Sa1=0; Sa2=1; Sa1P=1; Sa2P=0;
%             Sb1=0; Sb2=0; Sb1P=1; Sb2P=1;
%             Sc1=0; Sc2=1; Sc1P=1; Sc2P=0;        
%             pause(Ta/2);
%             Sa1=0; Sa2=0; Sa1P=1; Sa2P=1;
%             Sb1=0; Sb2=0; Sb1P=1; Sb2P=1;
%             Sc1=0; Sc2=1; Sc1P=1; Sc2P=0;
%             pause(Tc/2);
%             Sa1=0; Sa2=1; Sa1P=1; Sa2P=0;
%             Sb1=0; Sb2=0; Sb1P=1; Sb2P=1;
%             Sc1=0; Sc2=1; Sc1P=1; Sc2P=0;        
%             pause(Ta/2);
%             Sa1=0; Sa2=1; Sa1P=1; Sa2P=0;
%             Sb1=0; Sb2=0; Sb1P=1; Sb2P=1;
%             Sc1=1; Sc2=1; Sc1P=0; Sc2P=0;
%             pause(Tb/2);
%             Sa1=0; Sa2=1; Sa1P=1; Sa2P=0;
%             Sb1=0; Sb2=1; Sb1P=1; Sb2P=0;
%             Sc1=1; Sc2=1; Sc1P=0; Sc2P=0;
%             pause(Tc/4);
%         end
%         if angle>=3*pi/2 %then 2b
%             Sa1=1; Sa2=1; Sa1P=0; Sa2P=0;
%             Sb1=0; Sb2=1; Sb1P=1; Sb2P=0;
%             Sc1=1; Sc2=1; Sc1P=0; Sc2P=0;
%             pause(Tc/4);
%             Sa1=0; Sa2=1; Sa1P=1; Sa2P=0;
%             Sb1=0; Sb2=1; Sb1P=1; Sb2P=0;
%             Sc1=1; Sc2=1; Sc1P=0; Sc2P=0;
%             pause(Tb/2);
%             Sa1=0; Sa2=1; Sa1P=1; Sa2P=0;
%             Sb1=0; Sb2=0; Sb1P=1; Sb2P=1;
%             Sc1=1; Sc2=1; Sc1P=0; Sc2P=0;
%             pause(Ta/2);
%             Sa1=0; Sa2=1; Sa1P=1; Sa2P=0;
%             Sb1=0; Sb2=0; Sb1P=1; Sb2P=1;
%             Sc1=0; Sc2=1; Sc1P=1; Sc2P=0;
%             pause(Tc/2);
%             Sa1=0; Sa2=1; Sa1P=1; Sa2P=0;
%             Sb1=0; Sb2=0; Sb1P=1; Sb2P=1;
%             Sc1=1; Sc2=1; Sc1P=0; Sc2P=0;
%             pause(Ta/2);
%             Sa1=0; Sa2=1; Sa1P=1; Sa2P=0;
%             Sb1=0; Sb2=1; Sb1P=1; Sb2P=0;
%             Sc1=1; Sc2=1; Sc1P=0; Sc2P=0;
%             pause(Tb/2);
%             Sa1=1; Sa2=1; Sa1P=0; Sa2P=0;
%             Sb1=0; Sb2=1; Sb1P=1; Sb2P=0;
%             Sc1=1; Sc2=1; Sc1P=0; Sc2P=0;
%             pause(Tc/4);               
%         end
%     end
%     while(rgn4)
%          Sa1=1; Sa2=1; Sa1P=0; Sa2P=0; 
%          Sb1=0; Sb2=1; Sb1P=1; Sb2P=0;
%          Sc1=1; Sc2=1; Sc1P=0; Sc2P=0;
%          pause(Tc/4);
%          Sa1=1; Sa2=1; Sa1P=0; Sa2P=0;
%          Sb1=0; Sb2=0; Sb1P=1; Sb2P=1;
%          Sc1=1; Sc2=1; Sc1P=0; Sc2P=0;
%          pause(Tb/2);
%          Sa1=0; Sa2=1; Sa1P=1; Sa2P=0;
%          Sb1=0; Sb2=0; Sb1P=1; Sb2P=1;
%          Sc1=1; Sc2=1; Sc1P=0; Sc2P=0;
%          pause(Ta/2);
%          Sa1=0; Sa2=1; Sa1P=1; Sa2P=0;
%          Sb1=0; Sb2=0; Sb1P=1; Sb2P=1;
%          Sc1=0; Sc2=1; Sc1P=1; Sc2P=0;
%          pause(Tc/2);
%          Sa1=0; Sa2=1; Sa1P=1; Sa2P=0;
%          Sb1=0; Sb2=0; Sb1P=1; Sb2P=1;
%          Sc1=1; Sc2=1; Sc1P=0; Sc2P=0;
%          pause(Ta/2);
%          Sa1=1; Sa2=1; Sa1P=0; Sa2P=0;
%          Sb1=0; Sb2=0; Sb1P=1; Sb2P=1;
%          Sc1=1; Sc2=1; Sc1P=0; Sc2P=0;
%          pause(Tb/2);
%          Sa1=1; Sa2=1; Sa1P=0; Sa2P=0; 
%          Sb1=0; Sb2=1; Sb1P=1; Sb2P=0;
%          Sc1=1; Sc2=1; Sc1P=0; Sc2P=0;
%          pause(Tc/4);
%     end
%     
% end
% while(Sector6)
%     while(rgn3)
%         Sa1=1; Sa2=1; Sa1P=0; Sa2P=0;
%         Sb1=0; Sb2=1; Sb1P=1; Sb2P=0;
%         Sc1=1; Sc2=1; Sc1P=0; Sc2P=0;
%         pause(Tc/4);
%         Sa1=1; Sa2=1; Sa1P=0; Sa2P=0;
%         Sb1=0; Sb2=0; Sb1P=1; Sb2P=1;
%         Sc1=1; Sc2=1; Sc1P=0; Sc2P=0;
%         pause(Tb/2);
%         Sa1=1; Sa2=1; Sa1P=0; Sa2P=0;
%         Sb1=0; Sb2=0; Sb1P=1; Sb2P=1;
%         Sc1=0; Sc2=1; Sc1P=1; Sc2P=0;
%         pause(Ta/2);
%         Sa1=0; Sa2=1; Sa1P=1; Sa2P=0;
%         Sb1=0; Sb2=0; Sb1P=1; Sb2P=1;
%         Sc1=0; Sc2=1; Sc1P=1; Sc2P=0;
%         pause(Tc/2);
%         Sa1=1; Sa2=1; Sa1P=0; Sa2P=0;
%         Sb1=0; Sb2=0; Sb1P=1; Sb2P=1;
%         Sc1=0; Sc2=1; Sc1P=1; Sc2P=0;
%         pause(Ta/2);
%         Sa1=1; Sa2=1; Sa1P=0; Sa2P=0;
%         Sb1=0; Sb2=0; Sb1P=1; Sb2P=1;
%         Sc1=1; Sc2=1; Sc1P=0; Sc2P=0;
%         pause(Tb/2);
%         Sa1=1; Sa2=1; Sa1P=0; Sa2P=0;
%         Sb1=0; Sb2=1; Sb1P=1; Sb2P=0;
%         Sc1=1; Sc2=1; Sc1P=0; Sc2P=0;
%         pause(Tc/4);
%     end
%     while(rgn2)
%         if angle<=11*pi/6 %then 2a
%             Sa1=1; Sa2=1; Sa1P=0; Sa2P=0;
%             Sb1=0; Sb2=1; Sb1P=1; Sb2P=0;
%             Sc1=1; Sc2=1; Sc1P=0; Sc2P=0;
%             pause(Tc/4);
%             Sa1=1; Sa2=1; Sa1P=0; Sa2P=0;
%             Sb1=0; Sb2=1; Sb1P=1; Sb2P=0;
%             Sc1=0; Sc2=1; Sc1P=1; Sc2P=0;
%             pause(Tb/2);
%             Sa1=1; Sa2=1; Sa1P=0; Sa2P=0;
%             Sb1=0; Sb2=0; Sb1P=1; Sb2P=1;
%             Sc1=0; Sc2=1; Sc1P=1; Sc2P=0;
%             pause(Ta/2);
%             Sa1=0; Sa2=1; Sa1P=1; Sa2P=0;
%             Sb1=0; Sb2=0; Sb1P=1; Sb2P=1;
%             Sc1=0; Sc2=1; Sc1P=1; Sc2P=0;
%             pause(Tc/2);
%             Sa1=1; Sa2=1; Sa1P=0; Sa2P=0;
%             Sb1=0; Sb2=0; Sb1P=1; Sb2P=1;
%             Sc1=0; Sc2=1; Sc1P=1; Sc2P=0;
%             pause(Ta/2);
%             Sa1=1; Sa2=1; Sa1P=0; Sa2P=0;
%             Sb1=0; Sb2=1; Sb1P=1; Sb2P=0;
%             Sc1=0; Sc2=1; Sc1P=1; Sc2P=0;
%             pause(Tb/2); 
%             Sa1=1; Sa2=1; Sa1P=0; Sa2P=0;
%             Sb1=0; Sb2=1; Sb1P=1; Sb2P=0;
%             Sc1=1; Sc2=1; Sc1P=0; Sc2P=0;
%             pause(Tc/4);
%         end
%         if angle>=11*pi/6 %then 2b
%             Sa1=1; Sa2=1; Sa1P=0; Sa2P=0;
%             Sb1=0; Sb2=1; Sb1P=1; Sb2P=0;
%             Sc1=0; Sc2=1; Sc1P=1; Sc2P=0;
%             pause(Tc/4);
%             Sa1=1; Sa2=1; Sa1P=0; Sa2P=0;
%             Sb1=0; Sb2=0; Sb1P=1; Sb2P=1;
%             Sc1=0; Sc2=1; Sc1P=1; Sc2P=0;
%             pause(Tb/2);
%             Sa1=0; Sa2=1; Sa1P=1; Sa2P=0;
%             Sb1=0; Sb2=0; Sb1P=1; Sb2P=1;
%             Sc1=0; Sc2=1; Sc1P=1; Sc2P=0;
%             pause(Ta/2);
%             Sa1=0; Sa2=1; Sa1P=1; Sa2P=0;
%             Sb1=0; Sb2=0; Sb1P=1; Sb2P=1;
%             Sc1=0; Sc2=0; Sc1P=1; Sc2P=1;
%             pause(Tc/2);
%             Sa1=0; Sa2=1; Sa1P=1; Sa2P=0;
%             Sb1=0; Sb2=0; Sb1P=1; Sb2P=1;
%             Sc1=0; Sc2=1; Sc1P=1; Sc2P=0;
%             pause(Ta/2);
%             Sa1=1; Sa2=1; Sa1P=0; Sa2P=0;
%             Sb1=0; Sb2=0; Sb1P=1; Sb2P=1;
%             Sc1=0; Sc2=1; Sc1P=1; Sc2P=0;
%             pause(Tb/2);
%             Sa1=1; Sa2=1; Sa1P=0; Sa2P=0;
%             Sb1=0; Sb2=1; Sb1P=1; Sb2P=0;
%             Sc1=0; Sc2=1; Sc1P=1; Sc2P=0;
%             pause(Tc/4);
%         end
%     end
%     while(rgn4)
%         Sa1=1; Sa2=1; Sa1P=0; Sa2P=0;
%         Sb1=0; Sb2=1; Sb1P=1; Sb2P=0;
%         Sc1=0; Sc2=1; Sc1P=1; Sc2P=0;
%         pause(Tc/4);
%         Sa1=1; Sa2=1; Sa1P=0; Sa2P=0;
%         Sb1=0; Sb2=0; Sb1P=1; Sb2P=1;
%         Sc1=0; Sc2=1; Sc1P=1; Sc2P=0;
%         pause(Tb/2);
%         Sa1=1; Sa2=1; Sa1P=0; Sa2P=0;
%         Sb1=0; Sb2=0; Sb1P=1; Sb2P=1;
%         Sc1=0; Sc2=0; Sc1P=1; Sc2P=1;
%         pause(Ta/2);
%         Sa1=0; Sa2=1; Sa1P=1; Sa2P=0;
%         Sb1=0; Sb2=0; Sb1P=1; Sb2P=1;
%         Sc1=0; Sc2=0; Sc1P=1; Sc2P=1;
%         pause(Tc/2);
%         Sa1=1; Sa2=1; Sa1P=0; Sa2P=0;
%         Sb1=0; Sb2=0; Sb1P=1; Sb2P=1;
%         Sc1=0; Sc2=0; Sc1P=1; Sc2P=1;
%         pause(Ta/2);
%         Sa1=1; Sa2=1; Sa1P=0; Sa2P=0;
%         Sb1=0; Sb2=0; Sb1P=1; Sb2P=1;
%         Sc1=0; Sc2=1; Sc1P=1; Sc2P=0;
%         pause(Tb/2); 
%         Sa1=1; Sa2=1; Sa1P=0; Sa2P=0;
%         Sb1=0; Sb2=1; Sb1P=1; Sb2P=0;
%         Sc1=0; Sc2=1; Sc1P=1; Sc2P=0;
%         pause(Tc/4);
%     end
% end




%% test
output = Ts/(Ta+Tb+Tc);
%% duty cycles 
da = Ta/Ts;
db = Tb/Ts;
dc = Tc/Ts;
